simulink subsystem "LowLevelControllerSUB"  (R2023a)
settings: Solver=VariableStepAuto  StartTime=0.0  StopTime=10.0  RelTol=1e-3
undefined symbols (not defined in the file): km
settings Model: Creator=romav  LastModifiedBy=romav

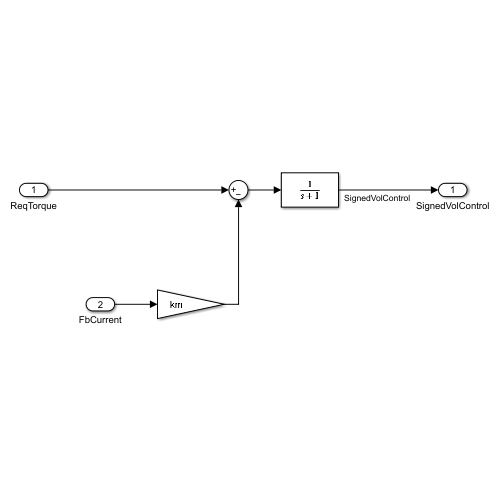
[thumbnail: Simulink's stored preview of the top-level diagram]
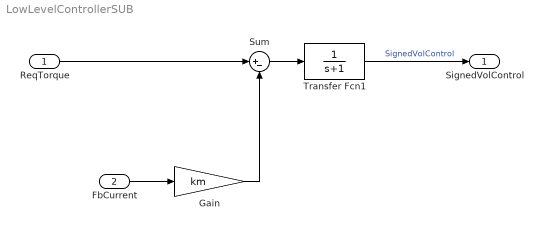
== system LowLevelControllerSUB ==
  ReqTorque : Inport
  FbCurrent : Inport  Port=2
  Gain : Gain  Gain=km
  Sum : Sum  Inputs=|+-
  Transfer Fcn1 : TransferFcn  Denominator=[1 1]
  SignedVolControl : Outport
  wires:
  Gain/1 -> Sum/2
  Transfer Fcn1/1 -> SignedVolControl/1  "SignedVolControl"
  Sum/1 -> Transfer Fcn1/1
  ReqTorque/1 -> Sum/1
  FbCurrent/1 -> Gain/1
